simulink library "halin"  (R2021b)
settings: Solver=VariableStepAuto  StartTime=0.0  StopTime=10.0  RelTol=1e-3
undefined symbols (not defined in the file): TRUE
libraries: FVT_lib x100, hcu_lib x41
(part 3 of 10)

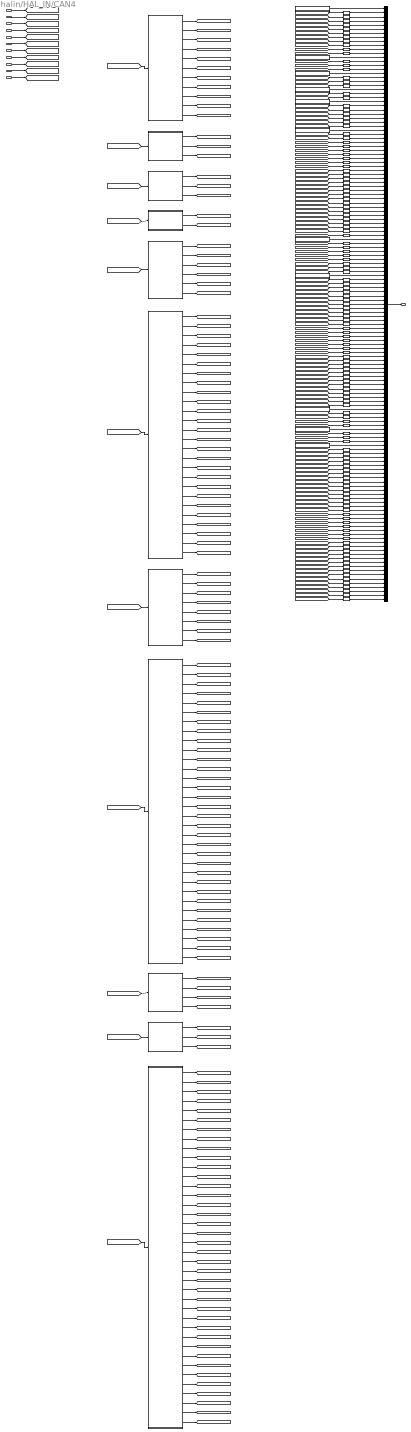
== system halin/HAL_IN/CAN4 ==
  DT_CAN4_SG_DKC1 : Inport
  DT_CAN4_SG_ZONE_DR_VCU : Inport  Port=2
  DT_CAN4_SG_ZONE_FR1 : Inport  Port=3
  DT_CAN4_SG_ZONE_FR_VCU : Inport  Port=4
  DT_CAN4_SG_zGW_APTC1 : Inport  Port=5
  DT_CAN4_SG_zGW_CANFr1 : Inport  Port=6
  DT_CAN4_SG_zGW_LINDr1 : Inport  Port=7
  DT_CAN4_SG_DKC2 : Inport  Port=8
  DT_CAN4_SG_Z24_C1000_0 : Inport  Port=9
  DT_CAN4_SG_Z24_CE100_0 : Inport  Port=10
  DT_CAN4_SG_ZONE_DR1 : Inport  Port=11
  DKC1 : Subsystem
  DKC2 : Subsystem
  UnitConverter{,1..7,9,25,31,33,35,37,39,41,43,45,47,49..50,58,60,62..67,70,72,74,76,78,80,82,84..88,90,99..100,102..104,120} (48 alike) : DataTypeConversion  OutDataTypeStr=uint8
  UnitConverter{8,10,17..20,23..24,26..29,51..52,55..57,68,98,101,105..107,109..110,112..113,115..116,118..119,121..135} (46 alike) : DataTypeConversion  OutDataTypeStr=boolean
  UnitConverter{14..16,21..22,30,32,34,36,38,40,42,44,46,48,53..54,59,61,69,71,73,75,77,79,81,83,89,91..96,108,111,114,117} (38 alike) : DataTypeConversion  OutDataTypeStr=single
  UnitConverter11 : DataTypeConversion  OutDataTypeStr=uint64
  UnitConverter12 : DataTypeConversion  OutDataTypeStr=uint64
  UnitConverter13 : DataTypeConversion  OutDataTypeStr=uint64
  UnitConverter97 : DataTypeConversion  OutDataTypeStr=uint16
  VHAL_CANMsgInvalidDKC1_flg : Subsystem  AncestorBlock=FVT_lib/hal/MsgTimeoutJudge_CAN_AUTOSAR
      mask help: MeasumentTrigerEvent
      mask Display: fprintf('MsgTimeoutJudge_CAN\nAUTOSAR');
  VHAL_CANMsgInvalidDKC2_flg : Subsystem  AncestorBlock=FVT_lib/hal/MsgTimeoutJudge_CAN_AUTOSAR
      mask help: MeasumentTrigerEvent
      mask Display: fprintf('MsgTimeoutJudge_CAN\nAUTOSAR');
  VHAL_CANMsgInvalidZ24C10000_flg : Subsystem  AncestorBlock=FVT_lib/hal/MsgTimeoutJudge_CAN_AUTOSAR
      mask help: MeasumentTrigerEvent
      mask Display: fprintf('MsgTimeoutJudge_CAN\nAUTOSAR');
  VHAL_CANMsgInvalidZ24CE1000_flg : Subsystem  AncestorBlock=FVT_lib/hal/MsgTimeoutJudge_CAN_AUTOSAR
      mask help: MeasumentTrigerEvent
      mask Display: fprintf('MsgTimeoutJudge_CAN\nAUTOSAR');
  VHAL_CANMsgInvalidZONEDR1_flg : Subsystem  AncestorBlock=FVT_lib/hal/MsgTimeoutJudge_CAN_AUTOSAR
      mask help: MeasumentTrigerEvent
      mask Display: fprintf('MsgTimeoutJudge_CAN\nAUTOSAR');
  VHAL_CANMsgInvalidZONEDRVCU_flg : Subsystem  AncestorBlock=FVT_lib/hal/MsgTimeoutJudge_CAN_AUTOSAR
      mask help: MeasumentTrigerEvent
      mask Display: fprintf('MsgTimeoutJudge_CAN\nAUTOSAR');
  VHAL_CANMsgInvalidZONEFR1_flg : Subsystem  AncestorBlock=FVT_lib/hal/MsgTimeoutJudge_CAN_AUTOSAR
      mask help: MeasumentTrigerEvent
      mask Display: fprintf('MsgTimeoutJudge_CAN\nAUTOSAR');
  VHAL_CANMsgInvalidZONEFRVCU_flg : Subsystem  AncestorBlock=FVT_lib/hal/MsgTimeoutJudge_CAN_AUTOSAR
      mask help: MeasumentTrigerEvent
      mask Display: fprintf('MsgTimeoutJudge_CAN\nAUTOSAR');
  VHAL_CANMsgInvalidzGWAPTC1_flg : Subsystem  AncestorBlock=FVT_lib/hal/MsgTimeoutJudge_CAN_AUTOSAR
      mask help: MeasumentTrigerEvent
      mask Display: fprintf('MsgTimeoutJudge_CAN\nAUTOSAR');
  VHAL_CANMsgInvalidzGWCANFr1_flg : Subsystem  AncestorBlock=FVT_lib/hal/MsgTimeoutJudge_CAN_AUTOSAR
      mask help: MeasumentTrigerEvent
      mask Display: fprintf('MsgTimeoutJudge_CAN\nAUTOSAR');
  VHAL_CANMsgInvalidzGWLINDr1_flg : Subsystem  AncestorBlock=FVT_lib/hal/MsgTimeoutJudge_CAN_AUTOSAR
      mask help: MeasumentTrigerEvent
      mask Display: fprintf('MsgTimeoutJudge_CAN\nAUTOSAR');
  Z24_C1000_0 : Subsystem
  Z24_CE100_0 : Subsystem
  ZONE_DR1 : Subsystem
  ZONE_DR_VCU : Subsystem
  ZONE_FR1 : Subsystem
  ZONE_FR_VCU : Subsystem
  bus_creator : BusCreator  Inputs=147
  zGW_APTC1 : Subsystem
  zGW_CANFr1 : Subsystem
  zGW_LINDr1 : Subsystem
  HAL_CAN4_outputs : Outport
  wires:
  DT_CAN4_SG_DKC1/1 -> [DT_CAN4_SG_DKC1]
  DT_CAN4_SG_ZONE_DR_VCU/1 -> [DT_CAN4_SG_ZONE_DR_VCU]
  DT_CAN4_SG_ZONE_FR1/1 -> [DT_CAN4_SG_ZONE_FR1]
  DT_CAN4_SG_ZONE_FR_VCU/1 -> [DT_CAN4_SG_ZONE_FR_VCU]
  DT_CAN4_SG_zGW_APTC1/1 -> [DT_CAN4_SG_zGW_APTC1]
  DT_CAN4_SG_zGW_CANFr1/1 -> [DT_CAN4_SG_zGW_CANFr1]
  DT_CAN4_SG_zGW_LINDr1/1 -> [DT_CAN4_SG_zGW_LINDr1]
  DT_CAN4_SG_DKC2/1 -> [DT_CAN4_SG_DKC2]
  DT_CAN4_SG_Z24_C1000_0/1 -> [DT_CAN4_SG_Z24_C1000_0]
  DT_CAN4_SG_Z24_CE100_0/1 -> [DT_CAN4_SG_Z24_CE100_0]
  DT_CAN4_SG_ZONE_DR1/1 -> [DT_CAN4_SG_ZONE_DR1]
  [DT_CAN4_SG_DKC1] -> DKC1/1(DT_CAN4_SG_DKC1)
  [DT_CAN4_SG_DKC2] -> DKC2/1(DT_CAN4_SG_DKC2)
  [DT_CAN4_SG_Z24_C1000_0] -> Z24_C1000_0/1(DT_CAN4_SG_Z24_C1000_0)
  [DT_CAN4_SG_Z24_CE100_0] -> Z24_CE100_0/1(DT_CAN4_SG_Z24_CE100_0)
  [DT_CAN4_SG_ZONE_DR1] -> ZONE_DR1/1(DT_CAN4_SG_ZONE_DR1)
  [DT_CAN4_SG_ZONE_DR_VCU] -> ZONE_DR_VCU/1(DT_CAN4_SG_ZONE_DR_VCU)
  [DT_CAN4_SG_ZONE_FR1] -> ZONE_FR1/1(DT_CAN4_SG_ZONE_FR1)
  [DT_CAN4_SG_ZONE_FR_VCU] -> ZONE_FR_VCU/1(DT_CAN4_SG_ZONE_FR_VCU)
  [DT_CAN4_SG_zGW_APTC1] -> zGW_APTC1/1(DT_CAN4_SG_zGW_APTC1)
  [DT_CAN4_SG_zGW_CANFr1] -> zGW_CANFr1/1(DT_CAN4_SG_zGW_CANFr1)
  [DT_CAN4_SG_zGW_LINDr1] -> zGW_LINDr1/1(DT_CAN4_SG_zGW_LINDr1)
  bus_creator/1 -> HAL_CAN4_outputs/1
  VHAL_CANMsgInvalidDKC1_flg/1(Out) -> bus_creator/1
  DKC1/1(VHAL_DKCReVehData_enum) -> [VHAL_DKCReVehData_enum]
  UnitConverter/1 -> bus_creator/2  "VHAL_DKCReVehData_enum"
  [VHAL_DKCReVehData_enum] -> UnitConverter/1
  DKC1/2(VHAL_PCommandToBCM_enum) -> [VHAL_PCommandToBCM_enum]
  UnitConverter1/1 -> bus_creator/3  "VHAL_PCommandToBCM_enum"
  [VHAL_PCommandToBCM_enum] -> UnitConverter1/1
  DKC1/3(VHAL_PCommandToPTG_enum) -> [VHAL_PCommandToPTG_enum]
  UnitConverter2/1 -> bus_creator/4  "VHAL_PCommandToPTG_enum"
  [VHAL_PCommandToPTG_enum] -> UnitConverter2/1
  DKC1/4(VHAL_PDKeyAreaLockUnlock_enum) -> [VHAL_PDKeyAreaLockUnlock_enum]
  UnitConverter3/1 -> bus_creator/5  "VHAL_PDKeyAreaLockUnlock_enum"
  [VHAL_PDKeyAreaLockUnlock_enum] -> UnitConverter3/1
  DKC1/5(VHAL_PDKeyAreaPS_enum) -> [VHAL_PDKeyAreaPS_enum]
  UnitConverter4/1 -> bus_creator/6  "VHAL_PDKeyAreaPS_enum"
  [VHAL_PDKeyAreaPS_enum] -> UnitConverter4/1
  DKC1/6(VHAL_PDKeyAreaPTG_enum) -> [VHAL_PDKeyAreaPTG_enum]
  UnitConverter5/1 -> bus_creator/7  "VHAL_PDKeyAreaPTG_enum"
  [VHAL_PDKeyAreaPTG_enum] -> UnitConverter5/1
  DKC1/7(VHAL_PDKeyWelcome_enum) -> [VHAL_PDKeyWelcome_enum]
  UnitConverter6/1 -> bus_creator/8  "VHAL_PDKeyWelcome_enum"
  [VHAL_PDKeyWelcome_enum] -> UnitConverter6/1
  DKC1/8(VHAL_PDkeyShowIVI_enum) -> [VHAL_PDkeyShowIVI_enum]
  UnitConverter7/1 -> bus_creator/9  "VHAL_PDkeyShowIVI_enum"
  [VHAL_PDkeyShowIVI_enum] -> UnitConverter7/1
  DKC1/9(VHAL_PKeyMiss_flg) -> [VHAL_PKeyMiss_flg]
  UnitConverter8/1 -> bus_creator/10  "VHAL_PKeyMiss_flg"
  [VHAL_PKeyMiss_flg] -> UnitConverter8/1
  DKC1/10(VHAL_PKeyMode_enum) -> [VHAL_PKeyMode_enum]
  UnitConverter9/1 -> bus_creator/11  "VHAL_PKeyMode_enum"
  [VHAL_PKeyMode_enum] -> UnitConverter9/1
  DKC1/11(VHAL_PUIDLowPower_flg) -> [VHAL_PUIDLowPower_flg]
  UnitConverter10/1 -> bus_creator/12  "VHAL_PUIDLowPower_flg"
  [VHAL_PUIDLowPower_flg] -> UnitConverter10/1
  VHAL_CANMsgInvalidDKC2_flg/1(Out) -> bus_creator/13
  DKC2/1(VHAL_EncryptionDATA063_enum) -> [VHAL_EncryptionDATA063_enum]
  UnitConverter11/1 -> bus_creator/14  "VHAL_EncryptionDATA063_enum"
  [VHAL_EncryptionDATA063_enum] -> UnitConverter11/1
  DKC2/2(VHAL_EncryptionDATA64127_enum) -> [VHAL_EncryptionDATA64127_enum]
  UnitConverter12/1 -> bus_creator/15  "VHAL_EncryptionDATA64127_enum"
  [VHAL_EncryptionDATA64127_enum] -> UnitConverter12/1
  DKC2/3(VHAL_RandomNumberX_enum) -> [VHAL_RandomNumberX_enum]
  UnitConverter13/1 -> bus_creator/16  "VHAL_RandomNumberX_enum"
  [VHAL_RandomNumberX_enum] -> UnitConverter13/1
  VHAL_CANMsgInvalidZ24C10000_flg/1(Out) -> bus_creator/17
  Z24_C1000_0/1(VHAL_Z24CHAAirPressureFC2Sta_KPa) -> [VHAL_Z24CHAAirPressureFC2Sta_KPa]
  UnitConverter14/1 -> bus_creator/18  "VHAL_Z24CHAAirPressureFC2Sta_KPa"
  [VHAL_Z24CHAAirPressureFC2Sta_KPa] -> UnitConverter14/1
  Z24_C1000_0/2(VHAL_Z24CHAAirPressurePC3Sta_KPa) -> [VHAL_Z24CHAAirPressurePC3Sta_KPa]
  UnitConverter15/1 -> bus_creator/19  "VHAL_Z24CHAAirPressurePC3Sta_KPa"
  [VHAL_Z24CHAAirPressurePC3Sta_KPa] -> UnitConverter15/1
  Z24_C1000_0/3(VHAL_Z24CHAAirPressureRC1Sta_KPa) -> [VHAL_Z24CHAAirPressureRC1Sta_KPa]
  UnitConverter16/1 -> bus_creator/20  "VHAL_Z24CHAAirPressureRC1Sta_KPa"
  [VHAL_Z24CHAAirPressureRC1Sta_KPa] -> UnitConverter16/1
  VHAL_CANMsgInvalidZ24CE1000_flg/1(Out) -> bus_creator/21
  Z24_CE100_0/1(VHAL_Z24BCMFWiperASSta_flg) -> [VHAL_Z24BCMFWiperASSta_flg]
  UnitConverter17/1 -> bus_creator/22  "VHAL_Z24BCMFWiperASSta_flg"
  [VHAL_Z24BCMFWiperASSta_flg] -> UnitConverter17/1
  Z24_CE100_0/2(VHAL_Z24BCMSeatBeltSWSta_flg) -> [VHAL_Z24BCMSeatBeltSWSta_flg]
  UnitConverter18/1 -> bus_creator/23  "VHAL_Z24BCMSeatBeltSWSta_flg"
  [VHAL_Z24BCMSeatBeltSWSta_flg] -> UnitConverter18/1
  VHAL_CANMsgInvalidZONEDR1_flg/1(Out) -> bus_creator/24
  ZONE_DR1/1(VHAL_DrLockSta_flg) -> [VHAL_DrLockSta_flg]
  UnitConverter19/1 -> bus_creator/25  "VHAL_DrLockSta_flg"
  [VHAL_DrLockSta_flg] -> UnitConverter19/1
  ZONE_DR1/2(VHAL_MIRRORFOLDSW_flg) -> [VHAL_MIRRORFOLDSW_flg]
  UnitConverter20/1 -> bus_creator/26  "VHAL_MIRRORFOLDSW_flg"
  [VHAL_MIRRORFOLDSW_flg] -> UnitConverter20/1
  ZONE_DR1/3(VHAL_RLTurnLampC_mA) -> [VHAL_RLTurnLampC_mA]
  UnitConverter21/1 -> bus_creator/27  "VHAL_RLTurnLampC_mA"
  [VHAL_RLTurnLampC_mA] -> UnitConverter21/1
  ZONE_DR1/4(VHAL_RRTurnLampC_mA) -> [VHAL_RRTurnLampC_mA]
  UnitConverter22/1 -> bus_creator/28  "VHAL_RRTurnLampC_mA"
  [VHAL_RRTurnLampC_mA] -> UnitConverter22/1
  ZONE_DR1/5(VHAL_RWiperAS_flg) -> [VHAL_RWiperAS_flg]
  UnitConverter23/1 -> bus_creator/29  "VHAL_RWiperAS_flg"
  [VHAL_RWiperAS_flg] -> UnitConverter23/1
  ZONE_DR1/6(VHAL_RWiperProtection_flg) -> [VHAL_RWiperProtection_flg]
  UnitConverter24/1 -> bus_creator/30  "VHAL_RWiperProtection_flg"
  [VHAL_RWiperProtection_flg] -> UnitConverter24/1
  VHAL_CANMsgInvalidZONEDRVCU_flg/1(Out) -> bus_creator/31
  ZONE_DR_VCU/1(VHAL_BlowerErr_enum) -> [VHAL_BlowerErr_enum]
  UnitConverter25/1 -> bus_creator/32  "VHAL_BlowerErr_enum"
  [VHAL_BlowerErr_enum] -> UnitConverter25/1
  ZONE_DR_VCU/2(VHAL_DrPMMLVOutPErrLmp_flg) -> [VHAL_DrPMMLVOutPErrLmp_flg]
  UnitConverter26/1 -> bus_creator/33  "VHAL_DrPMMLVOutPErrLmp_flg"
  [VHAL_DrPMMLVOutPErrLmp_flg] -> UnitConverter26/1
  ZONE_DR_VCU/3(VHAL_DrPMMSysErrLmp_flg) -> [VHAL_DrPMMSysErrLmp_flg]
  UnitConverter27/1 -> bus_creator/34  "VHAL_DrPMMSysErrLmp_flg"
  [VHAL_DrPMMSysErrLmp_flg] -> UnitConverter27/1
  ZONE_DR_VCU/4(VHAL_DrSCPSysErrLmp_flg) -> [VHAL_DrSCPSysErrLmp_flg]
  UnitConverter28/1 -> bus_creator/35  "VHAL_DrSCPSysErrLmp_flg"
  [VHAL_DrSCPSysErrLmp_flg] -> UnitConverter28/1
  ZONE_DR_VCU/5(VHAL_DrStdAErrSta_flg) -> [VHAL_DrStdAErrSta_flg]
  UnitConverter29/1 -> bus_creator/36  "VHAL_DrStdAErrSta_flg"
  [VHAL_DrStdAErrSta_flg] -> UnitConverter29/1
  ZONE_DR_VCU/6(VHAL_SolarL_W) -> [VHAL_SolarL_W]
  UnitConverter30/1 -> bus_creator/37  "VHAL_SolarL_W"
  [VHAL_SolarL_W] -> UnitConverter30/1
  ZONE_DR_VCU/7(VHAL_SolarLErr_enum) -> [VHAL_SolarLErr_enum]
  UnitConverter31/1 -> bus_creator/38  "VHAL_SolarLErr_enum"
  [VHAL_SolarLErr_enum] -> UnitConverter31/1
  ZONE_DR_VCU/8(VHAL_SolarR_W) -> [VHAL_SolarR_W]
  UnitConverter32/1 -> bus_creator/39  "VHAL_SolarR_W"
  [VHAL_SolarR_W] -> UnitConverter32/1
  ZONE_DR_VCU/9(VHAL_SolarRErr_enum) -> [VHAL_SolarRErr_enum]
  UnitConverter33/1 -> bus_creator/40  "VHAL_SolarRErr_enum"
  [VHAL_SolarRErr_enum] -> UnitConverter33/1
  ZONE_DR_VCU/10(VHAL_TFaceL_C) -> [VHAL_TFaceL_C]
  UnitConverter34/1 -> bus_creator/41  "VHAL_TFaceL_C"
  [VHAL_TFaceL_C] -> UnitConverter34/1
  ZONE_DR_VCU/11(VHAL_TFaceLErr_enum) -> [VHAL_TFaceLErr_enum]
  UnitConverter35/1 -> bus_creator/42  "VHAL_TFaceLErr_enum"
  [VHAL_TFaceLErr_enum] -> UnitConverter35/1
  ZONE_DR_VCU/12(VHAL_TFaceR_C) -> [VHAL_TFaceR_C]
  UnitConverter36/1 -> bus_creator/43  "VHAL_TFaceR_C"
  [VHAL_TFaceR_C] -> UnitConverter36/1
  ZONE_DR_VCU/13(VHAL_TFaceRErr_enum) -> [VHAL_TFaceRErr_enum]
  UnitConverter37/1 -> bus_creator/44  "VHAL_TFaceRErr_enum"
  [VHAL_TFaceRErr_enum] -> UnitConverter37/1
  ZONE_DR_VCU/14(VHAL_TFaceRr_C) -> [VHAL_TFaceRr_C]
  UnitConverter38/1 -> bus_creator/45  "VHAL_TFaceRr_C"
  [VHAL_TFaceRr_C] -> UnitConverter38/1
  ZONE_DR_VCU/15(VHAL_TFaceRrErr_enum) -> [VHAL_TFaceRrErr_enum]
  UnitConverter39/1 -> bus_creator/46  "VHAL_TFaceRrErr_enum"
  [VHAL_TFaceRrErr_enum] -> UnitConverter39/1
  ZONE_DR_VCU/16(VHAL_TFootL_C) -> [VHAL_TFootL_C]
  UnitConverter40/1 -> bus_creator/47  "VHAL_TFootL_C"
  [VHAL_TFootL_C] -> UnitConverter40/1
  ZONE_DR_VCU/17(VHAL_TFootLErr_enum) -> [VHAL_TFootLErr_enum]
  UnitConverter41/1 -> bus_creator/48  "VHAL_TFootLErr_enum"
  [VHAL_TFootLErr_enum] -> UnitConverter41/1
  ZONE_DR_VCU/18(VHAL_TFootR_C) -> [VHAL_TFootR_C]
  UnitConverter42/1 -> bus_creator/49  "VHAL_TFootR_C"
  [VHAL_TFootR_C] -> UnitConverter42/1
  ZONE_DR_VCU/19(VHAL_TFootRErr_enum) -> [VHAL_TFootRErr_enum]
  UnitConverter43/1 -> bus_creator/50  "VHAL_TFootRErr_enum"
  [VHAL_TFootRErr_enum] -> UnitConverter43/1
  ZONE_DR_VCU/20(VHAL_TFootRr_C) -> [VHAL_TFootRr_C]
  UnitConverter44/1 -> bus_creator/51  "VHAL_TFootRr_C"
  [VHAL_TFootRr_C] -> UnitConverter44/1
  ZONE_DR_VCU/21(VHAL_TFootRrErr_enum) -> [VHAL_TFootRrErr_enum]
  UnitConverter45/1 -> bus_creator/52  "VHAL_TFootRrErr_enum"
  [VHAL_TFootRrErr_enum] -> UnitConverter45/1
  ZONE_DR_VCU/22(VHAL_Tevap_C) -> [VHAL_Tevap_C]
  UnitConverter46/1 -> bus_creator/53  "VHAL_Tevap_C"
  [VHAL_Tevap_C] -> UnitConverter46/1
  ZONE_DR_VCU/23(VHAL_TevapErr_enum) -> [VHAL_TevapErr_enum]
  UnitConverter47/1 -> bus_creator/54  "VHAL_TevapErr_enum"
  [VHAL_TevapErr_enum] -> UnitConverter47/1
  ZONE_DR_VCU/24(VHAL_Tincar_C) -> [VHAL_Tincar_C]
  UnitConverter48/1 -> bus_creator/55  "VHAL_Tincar_C"
  [VHAL_Tincar_C] -> UnitConverter48/1
  ZONE_DR_VCU/25(VHAL_TincarErr_enum) -> [VHAL_TincarErr_enum]
  UnitConverter49/1 -> bus_creator/56  "VHAL_TincarErr_enum"
  [VHAL_TincarErr_enum] -> UnitConverter49/1
  ZONE_DR_VCU/26(VHAL_ZoneDrMalfunLevel_enum) -> [VHAL_ZoneDrMalfunLevel_enum]
  UnitConverter50/1 -> bus_creator/57  "VHAL_ZoneDrMalfunLevel_enum"
  [VHAL_ZoneDrMalfunLevel_enum] -> UnitConverter50/1
  VHAL_CANMsgInvalidZONEFR1_flg/1(Out) -> bus_creator/58
  ZONE_FR1/1(VHAL_ChargeInletLockSta_flg) -> [VHAL_ChargeInletLockSta_flg]
  UnitConverter51/1 -> bus_creator/59  "VHAL_ChargeInletLockSta_flg"
  [VHAL_ChargeInletLockSta_flg] -> UnitConverter51/1
  ZONE_FR1/2(VHAL_CompProEN_flg) -> [VHAL_CompProEN_flg]
  UnitConverter52/1 -> bus_creator/60  "VHAL_CompProEN_flg"
  [VHAL_CompProEN_flg] -> UnitConverter52/1
  ZONE_FR1/3(VHAL_FLTurnLampC_mA) -> [VHAL_FLTurnLampC_mA]
  UnitConverter53/1 -> bus_creator/61  "VHAL_FLTurnLampC_mA"
  [VHAL_FLTurnLampC_mA] -> UnitConverter53/1
  ZONE_FR1/4(VHAL_FRTurnLampC_mA) -> [VHAL_FRTurnLampC_mA]
  UnitConverter54/1 -> bus_creator/62  "VHAL_FRTurnLampC_mA"
  [VHAL_FRTurnLampC_mA] -> UnitConverter54/1
  ZONE_FR1/5(VHAL_FWiperAS_flg) -> [VHAL_FWiperAS_flg]
  UnitConverter55/1 -> bus_creator/63  "VHAL_FWiperAS_flg"
  [VHAL_FWiperAS_flg] -> UnitConverter55/1
  ZONE_FR1/6(VHAL_FWiperProtection_flg) -> [VHAL_FWiperProtection_flg]
  UnitConverter56/1 -> bus_creator/64  "VHAL_FWiperProtection_flg"
  [VHAL_FWiperProtection_flg] -> UnitConverter56/1
  ZONE_FR1/7(VHAL_TrailerCheck_flg) -> [VHAL_TrailerCheck_flg]
  UnitConverter57/1 -> bus_creator/65  "VHAL_TrailerCheck_flg"
  [VHAL_TrailerCheck_flg] -> UnitConverter57/1
  ZONE_FR1/8(VHAL_TrailerModeSta_enum) -> [VHAL_TrailerModeSta_enum]
  UnitConverter58/1 -> bus_creator/66  "VHAL_TrailerModeSta_enum"
  [VHAL_TrailerModeSta_enum] -> UnitConverter58/1
  VHAL_CANMsgInvalidZONEFRVCU_flg/1(Out) -> bus_creator/67
  ZONE_FR_VCU/1(VHAL_BatInTemp_C) -> [VHAL_BatInTemp_C]
  UnitConverter59/1 -> bus_creator/68  "VHAL_BatInTemp_C"
  [VHAL_BatInTemp_C] -> UnitConverter59/1
  ZONE_FR_VCU/2(VHAL_BatInTempErr_enum) -> [VHAL_BatInTempErr_enum]
  UnitConverter60/1 -> bus_creator/69  "VHAL_BatInTempErr_enum"
  [VHAL_BatInTempErr_enum] -> UnitConverter60/1
  ZONE_FR_VCU/3(VHAL_BatOutTemp_C) -> [VHAL_BatOutTemp_C]
  UnitConverter61/1 -> bus_creator/70  "VHAL_BatOutTemp_C"
  [VHAL_BatOutTemp_C] -> UnitConverter61/1
  ZONE_FR_VCU/4(VHAL_COMPErr_enum) -> [VHAL_COMPErr_enum]
  UnitConverter62/1 -> bus_creator/71  "VHAL_COMPErr_enum"
  [VHAL_COMPErr_enum] -> UnitConverter62/1
  ZONE_FR_VCU/5(VHAL_EACProtectEnable_enum) -> [VHAL_EACProtectEnable_enum]
  UnitConverter63/1 -> bus_creator/72  "VHAL_EACProtectEnable_enum"
  [VHAL_EACProtectEnable_enum] -> UnitConverter63/1
  ZONE_FR_VCU/6(VHAL_EWP3Err_enum) -> [VHAL_EWP3Err_enum]
  UnitConverter64/1 -> bus_creator/73  "VHAL_EWP3Err_enum"
  [VHAL_EWP3Err_enum] -> UnitConverter64/1
  ZONE_FR_VCU/7(VHAL_EXV1Err_enum) -> [VHAL_EXV1Err_enum]
  UnitConverter65/1 -> bus_creator/74  "VHAL_EXV1Err_enum"
  [VHAL_EXV1Err_enum] -> UnitConverter65/1
  ZONE_FR_VCU/8(VHAL_EXV2Err_enum) -> [VHAL_EXV2Err_enum]
  UnitConverter66/1 -> bus_creator/75  "VHAL_EXV2Err_enum"
  [VHAL_EXV2Err_enum] -> UnitConverter66/1
  ZONE_FR_VCU/9(VHAL_FanErr_enum) -> [VHAL_FanErr_enum]
  UnitConverter67/1 -> bus_creator/76  "VHAL_FanErr_enum"
  [VHAL_FanErr_enum] -> UnitConverter67/1
  ZONE_FR_VCU/10(VHAL_FrPMMLimpHomeActReq_flg) -> [VHAL_FrPMMLimpHomeActReq_flg]
  UnitConverter68/1 -> bus_creator/77  "VHAL_FrPMMLimpHomeActReq_flg"
  [VHAL_FrPMMLimpHomeActReq_flg] -> UnitConverter68/1
  ZONE_FR_VCU/11(VHAL_MotorInTemp_C) -> [VHAL_MotorInTemp_C]
  UnitConverter69/1 -> bus_creator/78  "VHAL_MotorInTemp_C"
  [VHAL_MotorInTemp_C] -> UnitConverter69/1
  ZONE_FR_VCU/12(VHAL_MotorInTempErr_enum) -> [VHAL_MotorInTempErr_enum]
  UnitConverter70/1 -> bus_creator/79  "VHAL_MotorInTempErr_enum"
  [VHAL_MotorInTempErr_enum] -> UnitConverter70/1
  ZONE_FR_VCU/13(VHAL_MotorOutTemp_C) -> [VHAL_MotorOutTemp_C]
  UnitConverter71/1 -> bus_creator/80  "VHAL_MotorOutTemp_C"
  [VHAL_MotorOutTemp_C] -> UnitConverter71/1
  ZONE_FR_VCU/14(VHAL_MotorOutTempErr_enum) -> [VHAL_MotorOutTempErr_enum]
  UnitConverter72/1 -> bus_creator/81  "VHAL_MotorOutTempErr_enum"
  [VHAL_MotorOutTempErr_enum] -> UnitConverter72/1
  ZONE_FR_VCU/15(VHAL_PTHighP_KPa) -> [VHAL_PTHighP_KPa]
  UnitConverter73/1 -> bus_creator/82  "VHAL_PTHighP_KPa"
  [VHAL_PTHighP_KPa] -> UnitConverter73/1
  ZONE_FR_VCU/16(VHAL_PTHighPErr_enum) -> [VHAL_PTHighPErr_enum]
  UnitConverter74/1 -> bus_creator/83  "VHAL_PTHighPErr_enum"
  [VHAL_PTHighPErr_enum] -> UnitConverter74/1
  ZONE_FR_VCU/17(VHAL_PTHighTact_C) -> [VHAL_PTHighTact_C]
  UnitConverter75/1 -> bus_creator/84  "VHAL_PTHighTact_C"
  [VHAL_PTHighTact_C] -> UnitConverter75/1
  ZONE_FR_VCU/18(VHAL_PTHighTactErr_enum) -> [VHAL_PTHighTactErr_enum]
  UnitConverter76/1 -> bus_creator/85  "VHAL_PTHighTactErr_enum"
  [VHAL_PTHighTactErr_enum] -> UnitConverter76/1
  ZONE_FR_VCU/19(VHAL_PTLowP1_KPa) -> [VHAL_PTLowP1_KPa]
  UnitConverter77/1 -> bus_creator/86  "VHAL_PTLowP1_KPa"
  [VHAL_PTLowP1_KPa] -> UnitConverter77/1
  ZONE_FR_VCU/20(VHAL_PTLowP1Err_enum) -> [VHAL_PTLowP1Err_enum]
  UnitConverter78/1 -> bus_creator/87  "VHAL_PTLowP1Err_enum"
  [VHAL_PTLowP1Err_enum] -> UnitConverter78/1
  ZONE_FR_VCU/21(VHAL_PTLowP2_KPa) -> [VHAL_PTLowP2_KPa]
  UnitConverter79/1 -> bus_creator/88  "VHAL_PTLowP2_KPa"
  [VHAL_PTLowP2_KPa] -> UnitConverter79/1
  ZONE_FR_VCU/22(VHAL_PTLowP2Err_enum) -> [VHAL_PTLowP2Err_enum]
  UnitConverter80/1 -> bus_creator/89  "VHAL_PTLowP2Err_enum"
  [VHAL_PTLowP2Err_enum] -> UnitConverter80/1
  ZONE_FR_VCU/23(VHAL_PTLowT1_C) -> [VHAL_PTLowT1_C]
  UnitConverter81/1 -> bus_creator/90  "VHAL_PTLowT1_C"
  [VHAL_PTLowT1_C] -> UnitConverter81/1
  ZONE_FR_VCU/24(VHAL_PTLowT1Err_enum) -> [VHAL_PTLowT1Err_enum]
  UnitConverter82/1 -> bus_creator/91  "VHAL_PTLowT1Err_enum"
  [VHAL_PTLowT1Err_enum] -> UnitConverter82/1
  ZONE_FR_VCU/25(VHAL_PTLowT2_C) -> [VHAL_PTLowT2_C]
  UnitConverter83/1 -> bus_creator/92  "VHAL_PTLowT2_C"
  [VHAL_PTLowT2_C] -> UnitConverter83/1
  ZONE_FR_VCU/26(VHAL_PTLowT2Err_enum) -> [VHAL_PTLowT2Err_enum]
  UnitConverter84/1 -> bus_creator/93  "VHAL_PTLowT2Err_enum"
  [VHAL_PTLowT2Err_enum] -> UnitConverter84/1
  ZONE_FR_VCU/27(VHAL_SOTXVErr_enum) -> [VHAL_SOTXVErr_enum]
  UnitConverter85/1 -> bus_creator/94  "VHAL_SOTXVErr_enum"
  [VHAL_SOTXVErr_enum] -> UnitConverter85/1
  ZONE_FR_VCU/28(VHAL_SOV1Err_enum) -> [VHAL_SOV1Err_enum]
  UnitConverter86/1 -> bus_creator/95  "VHAL_SOV1Err_enum"
  [VHAL_SOV1Err_enum] -> UnitConverter86/1
  ZONE_FR_VCU/29(VHAL_SOV2Err_enum) -> [VHAL_SOV2Err_enum]
  UnitConverter87/1 -> bus_creator/96  "VHAL_SOV2Err_enum"
  [VHAL_SOV2Err_enum] -> UnitConverter87/1
  ZONE_FR_VCU/30(VHAL_SOV3Err_enum) -> [VHAL_SOV3Err_enum]
  UnitConverter88/1 -> bus_creator/97  "VHAL_SOV3Err_enum"
  [VHAL_SOV3Err_enum] -> UnitConverter88/1
  ZONE_FR_VCU/31(VHAL_Tamb_C) -> [VHAL_Tamb_C]
  UnitConverter89/1 -> bus_creator/98  "VHAL_Tamb_C"
  [VHAL_Tamb_C] -> UnitConverter89/1
  ZONE_FR_VCU/32(VHAL_TambErr_enum) -> [VHAL_TambErr_enum]
  UnitConverter90/1 -> bus_creator/99  "VHAL_TambErr_enum"
  [VHAL_TambErr_enum] -> UnitConverter90/1
  VHAL_CANMsgInvalidzGWAPTC1_flg/1(Out) -> bus_creator/100
  zGW_APTC1/1(VHAL_FrntPTCLeActHeatPwr_W) -> [VHAL_FrntPTCLeActHeatPwr_W]
  UnitConverter91/1 -> bus_creator/101  "VHAL_FrntPTCLeActHeatPwr_W"
  [VHAL_FrntPTCLeActHeatPwr_W] -> UnitConverter91/1
  zGW_APTC1/2(VHAL_FrntPTCRearLeActHeatPwr_W) -> [VHAL_FrntPTCRearLeActHeatPwr_W]
  UnitConverter92/1 -> bus_creator/102  "VHAL_FrntPTCRearLeActHeatPwr_W"
  [VHAL_FrntPTCRearLeActHeatPwr_W] -> UnitConverter92/1
  zGW_APTC1/3(VHAL_FrntPTCRearRiActHeatPwr_W) -> [VHAL_FrntPTCRearRiActHeatPwr_W]
  UnitConverter93/1 -> bus_creator/103  "VHAL_FrntPTCRearRiActHeatPwr_W"
  [VHAL_FrntPTCRearRiActHeatPwr_W] -> UnitConverter93/1
  zGW_APTC1/4(VHAL_FrntPTCRiActHeatPwr_W) -> [VHAL_FrntPTCRiActHeatPwr_W]
  UnitConverter94/1 -> bus_creator/104  "VHAL_FrntPTCRiActHeatPwr_W"
  [VHAL_FrntPTCRiActHeatPwr_W] -> UnitConverter94/1
  VHAL_CANMsgInvalidzGWCANFr1_flg/1(Out) -> bus_creator/105
  zGW_CANFr1/1(VHAL_COMPActualPwr_W) -> [VHAL_COMPActualPwr_W]
  UnitConverter95/1 -> bus_creator/106  "VHAL_COMPActualPwr_W"
  [VHAL_COMPActualPwr_W] -> UnitConverter95/1
  zGW_CANFr1/2(VHAL_COMPStatorSpd_rpm) -> [VHAL_COMPStatorSpd_rpm]
  UnitConverter96/1 -> bus_creator/107  "VHAL_COMPStatorSpd_rpm"
  [VHAL_COMPStatorSpd_rpm] -> UnitConverter96/1
  zGW_CANFr1/3(VHAL_PTCActuPwrHSC6_enum) -> [VHAL_PTCActuPwrHSC6_enum]
  UnitConverter97/1 -> bus_creator/108  "VHAL_PTCActuPwrHSC6_enum"
  [VHAL_PTCActuPwrHSC6_enum] -> UnitConverter97/1
  VHAL_CANMsgInvalidzGWLINDr1_flg/1(Out) -> bus_creator/109
  zGW_LINDr1/1(VHAL_CSWDimSw_flg) -> [VHAL_CSWDimSw_flg]
  UnitConverter98/1 -> bus_creator/110  "VHAL_CSWDimSw_flg"
  [VHAL_CSWDimSw_flg] -> UnitConverter98/1
  zGW_LINDr1/2(VHAL_CSWFWasSwSta_enum) -> [VHAL_CSWFWasSwSta_enum]
  UnitConverter99/1 -> bus_creator/111  "VHAL_CSWFWasSwSta_enum"
  [VHAL_CSWFWasSwSta_enum] -> UnitConverter99/1
  zGW_LINDr1/3(VHAL_CSWFWipSwSta_enum) -> [VHAL_CSWFWipSwSta_enum]
  UnitConverter100/1 -> bus_creator/112  "VHAL_CSWFWipSwSta_enum"
  [VHAL_CSWFWipSwSta_enum] -> UnitConverter100/1
  zGW_LINDr1/4(VHAL_CSWPassSWSta_flg) -> [VHAL_CSWPassSWSta_flg]
  UnitConverter101/1 -> bus_creator/113  "VHAL_CSWPassSWSta_flg"
  [VHAL_CSWPassSWSta_flg] -> UnitConverter101/1
  zGW_LINDr1/5(VHAL_CSWRWasSWSta_enum) -> [VHAL_CSWRWasSWSta_enum]
  UnitConverter102/1 -> bus_creator/114  "VHAL_CSWRWasSWSta_enum"
  [VHAL_CSWRWasSWSta_enum] -> UnitConverter102/1
  zGW_LINDr1/6(VHAL_CSWRWipIntSwSta_enum) -> [VHAL_CSWRWipIntSwSta_enum]
  UnitConverter103/1 -> bus_creator/115  "VHAL_CSWRWipIntSwSta_enum"
  [VHAL_CSWRWipIntSwSta_enum] -> UnitConverter103/1
  zGW_LINDr1/7(VHAL_CSWTurnSwSta_enum) -> [VHAL_CSWTurnSwSta_enum]
  UnitConverter104/1 -> bus_creator/116  "VHAL_CSWTurnSwSta_enum"
  [VHAL_CSWTurnSwSta_enum] -> UnitConverter104/1
  zGW_LINDr1/8(VHAL_FAPWL01LINResponseError_flg) -> [VHAL_FAPWL01LINResponseError_flg]
  UnitConverter105/1 -> bus_creator/117  "VHAL_FAPWL01LINResponseError_flg"
  [VHAL_FAPWL01LINResponseError_flg] -> UnitConverter105/1
  zGW_LINDr1/9(VHAL_LDrvMotorRelayError_flg) -> [VHAL_LDrvMotorRelayError_flg]
  UnitConverter106/1 -> bus_creator/118  "VHAL_LDrvMotorRelayError_flg"
  [VHAL_LDrvMotorRelayError_flg] -> UnitConverter106/1
  zGW_LINDr1/10(VHAL_LDrvMotorRippleError_flg) -> [VHAL_LDrvMotorRippleError_flg]
  UnitConverter107/1 -> bus_creator/119  "VHAL_LDrvMotorRippleError_flg"
  [VHAL_LDrvMotorRippleError_flg] -> UnitConverter107/1
  zGW_LINDr1/11(VHAL_LDrvValWdwOpened_pct) -> [VHAL_LDrvValWdwOpened_pct]
  UnitConverter108/1 -> bus_creator/120  "VHAL_LDrvValWdwOpened_pct"
  [VHAL_LDrvValWdwOpened_pct] -> UnitConverter108/1
  zGW_LINDr1/12(VHAL_LPasMotorRelayError_flg) -> [VHAL_LPasMotorRelayError_flg]
  UnitConverter109/1 -> bus_creator/121  "VHAL_LPasMotorRelayError_flg"
  [VHAL_LPasMotorRelayError_flg] -> UnitConverter109/1
  zGW_LINDr1/13(VHAL_LPasMotorRippleError_flg) -> [VHAL_LPasMotorRippleError_flg]
  UnitConverter110/1 -> bus_creator/122  "VHAL_LPasMotorRippleError_flg"
  [VHAL_LPasMotorRippleError_flg] -> UnitConverter110/1
  zGW_LINDr1/14(VHAL_LPasValWdwOpened_pct) -> [VHAL_LPasValWdwOpened_pct]
  UnitConverter111/1 -> bus_creator/123  "VHAL_LPasValWdwOpened_pct"
  [VHAL_LPasValWdwOpened_pct] -> UnitConverter111/1
  zGW_LINDr1/15(VHAL_LRLDMotorRelayError_flg) -> [VHAL_LRLDMotorRelayError_flg]
  UnitConverter112/1 -> bus_creator/124  "VHAL_LRLDMotorRelayError_flg"
  [VHAL_LRLDMotorRelayError_flg] -> UnitConverter112/1
  zGW_LINDr1/16(VHAL_LRLDMotorRippleError_flg) -> [VHAL_LRLDMotorRippleError_flg]
  UnitConverter113/1 -> bus_creator/125  "VHAL_LRLDMotorRippleError_flg"
  [VHAL_LRLDMotorRippleError_flg] -> UnitConverter113/1
  zGW_LINDr1/17(VHAL_LRLDValWdwOpened_pct) -> [VHAL_LRLDValWdwOpened_pct]
  UnitConverter114/1 -> bus_creator/126  "VHAL_LRLDValWdwOpened_pct"
  [VHAL_LRLDValWdwOpened_pct] -> UnitConverter114/1
  zGW_LINDr1/18(VHAL_LRRDMotorRelayError_flg) -> [VHAL_LRRDMotorRelayError_flg]
  UnitConverter115/1 -> bus_creator/127  "VHAL_LRRDMotorRelayError_flg"
  [VHAL_LRRDMotorRelayError_flg] -> UnitConverter115/1
  zGW_LINDr1/19(VHAL_LRRDMotorRippleError_flg) -> [VHAL_LRRDMotorRippleError_flg]
  UnitConverter116/1 -> bus_creator/128  "VHAL_LRRDMotorRippleError_flg"
  [VHAL_LRRDMotorRippleError_flg] -> UnitConverter116/1
  zGW_LINDr1/20(VHAL_LRRDValWdwOpened_pct) -> [VHAL_LRRDValWdwOpened_pct]
  UnitConverter117/1 -> bus_creator/129  "VHAL_LRRDValWdwOpened_pct"
  [VHAL_LRRDValWdwOpened_pct] -> UnitConverter117/1
  zGW_LINDr1/21(VHAL_RAPWL01LINResponseError_flg) -> [VHAL_RAPWL01LINResponseError_flg]
  UnitConverter118/1 -> bus_creator/130  "VHAL_RAPWL01LINResponseError_flg"
  [VHAL_RAPWL01LINResponseError_flg] -> UnitConverter118/1
  zGW_LINDr1/22(VHAL_RLSLampSta_flg) -> [VHAL_RLSLampSta_flg]
  UnitConverter119/1 -> bus_creator/131  "VHAL_RLSLampSta_flg"
  [VHAL_RLSLampSta_flg] -> UnitConverter119/1
  zGW_LINDr1/23(VHAL_RLSRainSnrWiperCmd_enum) -> [VHAL_RLSRainSnrWiperCmd_enum]
  UnitConverter120/1 -> bus_creator/132  "VHAL_RLSRainSnrWiperCmd_enum"
  [VHAL_RLSRainSnrWiperCmd_enum] -> UnitConverter120/1
  zGW_LINDr1/24(VHAL_SWCACCSta_flg) -> [VHAL_SWCACCSta_flg]
  UnitConverter121/1 -> bus_creator/133  "VHAL_SWCACCSta_flg"
  [VHAL_SWCACCSta_flg] -> UnitConverter121/1
  zGW_LINDr1/25(VHAL_SWCCANCELSta_flg) -> [VHAL_SWCCANCELSta_flg]
  UnitConverter122/1 -> bus_creator/134  "VHAL_SWCCANCELSta_flg"
  [VHAL_SWCCANCELSta_flg] -> UnitConverter122/1
  zGW_LINDr1/26(VHAL_SWCDistanceSta_flg) -> [VHAL_SWCDistanceSta_flg]
  UnitConverter123/1 -> bus_creator/135  "VHAL_SWCDistanceSta_flg"
  [VHAL_SWCDistanceSta_flg] -> UnitConverter123/1
  zGW_LINDr1/27(VHAL_SWCDownSta_flg) -> [VHAL_SWCDownSta_flg]
  UnitConverter124/1 -> bus_creator/136  "VHAL_SWCDownSta_flg"
  [VHAL_SWCDownSta_flg] -> UnitConverter124/1
  zGW_LINDr1/28(VHAL_SWCLKASta_flg) -> [VHAL_SWCLKASta_flg]
  UnitConverter125/1 -> bus_creator/137  "VHAL_SWCLKASta_flg"
  [VHAL_SWCLKASta_flg] -> UnitConverter125/1
  zGW_LINDr1/29(VHAL_SWCLeftSta_flg) -> [VHAL_SWCLeftSta_flg]
  UnitConverter126/1 -> bus_creator/138  "VHAL_SWCLeftSta_flg"
  [VHAL_SWCLeftSta_flg] -> UnitConverter126/1
  zGW_LINDr1/30(VHAL_SWCRegenUp_flg) -> [VHAL_SWCRegenUp_flg]
  UnitConverter127/1 -> bus_creator/139  "VHAL_SWCRegenUp_flg"
  [VHAL_SWCRegenUp_flg] -> UnitConverter127/1
  zGW_LINDr1/31(VHAL_SWCResUpSta_flg) -> [VHAL_SWCResUpSta_flg]
  UnitConverter128/1 -> bus_creator/140  "VHAL_SWCResUpSta_flg"
  [VHAL_SWCResUpSta_flg] -> UnitConverter128/1
  zGW_LINDr1/32(VHAL_SWCRightSta_flg) -> [VHAL_SWCRightSta_flg]
  UnitConverter129/1 -> bus_creator/141  "VHAL_SWCRightSta_flg"
  [VHAL_SWCRightSta_flg] -> UnitConverter129/1
  zGW_LINDr1/33(VHAL_SWCSetdownSta_flg) -> [VHAL_SWCSetdownSta_flg]
  UnitConverter130/1 -> bus_creator/142  "VHAL_SWCSetdownSta_flg"
  [VHAL_SWCSetdownSta_flg] -> UnitConverter130/1
  zGW_LINDr1/34(VHAL_SWCTripSta_flg) -> [VHAL_SWCTripSta_flg]
  UnitConverter131/1 -> bus_creator/143  "VHAL_SWCTripSta_flg"
  [VHAL_SWCTripSta_flg] -> UnitConverter131/1
  zGW_LINDr1/35(VHAL_SWCUndefinedSta_flg) -> [VHAL_SWCUndefinedSta_flg]
  UnitConverter132/1 -> bus_creator/144  "VHAL_SWCUndefinedSta_flg"
  [VHAL_SWCUndefinedSta_flg] -> UnitConverter132/1
  zGW_LINDr1/36(VHAL_SWCUpSta_flg) -> [VHAL_SWCUpSta_flg]
  UnitConverter133/1 -> bus_creator/145  "VHAL_SWCUpSta_flg"
  [VHAL_SWCUpSta_flg] -> UnitConverter133/1
  zGW_LINDr1/37(VHAL_SWCVRSta_flg) -> [VHAL_SWCVRSta_flg]
  UnitConverter134/1 -> bus_creator/146  "VHAL_SWCVRSta_flg"
  [VHAL_SWCVRSta_flg] -> UnitConverter134/1
  zGW_LINDr1/38(VHAL_SWCmodeSta_flg) -> [VHAL_SWCmodeSta_flg]
  UnitConverter135/1 -> bus_creator/147  "VHAL_SWCmodeSta_flg"
  [VHAL_SWCmodeSta_flg] -> UnitConverter135/1

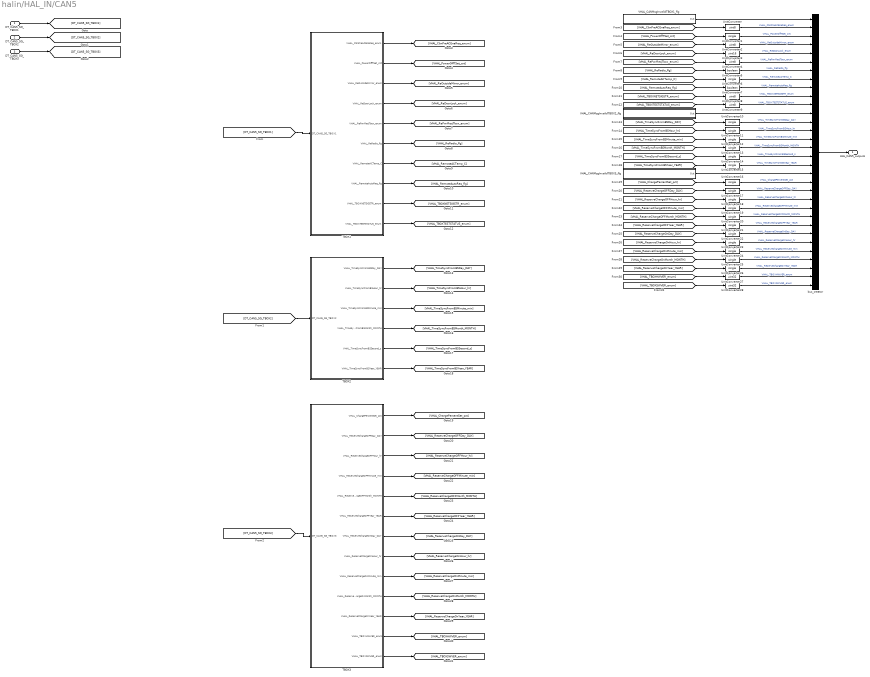
== system halin/HAL_IN/CAN5 ==
  DT_CAN5_SG_TBOX1 : Inport
  DT_CAN5_SG_TBOX2 : Inport  Port=2
  DT_CAN5_SG_TBOX3 : Inport  Port=3
  TBOX1 : Subsystem
  TBOX2 : Subsystem
  TBOX3 : Subsystem
  UnitConverter{,2,4,8..9} (5 alike) : DataTypeConversion  OutDataTypeStr=uint8
  UnitConverter{1,6,10..26} (19 alike) : DataTypeConversion  OutDataTypeStr=single
  UnitConverter27 : DataTypeConversion  OutDataTypeStr=uint32
  UnitConverter28 : DataTypeConversion  OutDataTypeStr=uint32
  UnitConverter3 : DataTypeConversion  OutDataTypeStr=uint16
  UnitConverter5 : DataTypeConversion  OutDataTypeStr=boolean
  UnitConverter7 : DataTypeConversion  OutDataTypeStr=boolean
  VHAL_CANMsgInvalidTBOX1_flg : Subsystem  AncestorBlock=FVT_lib/hal/MsgTimeoutJudge_CAN_AUTOSAR
      mask help: MeasumentTrigerEvent
      mask Display: fprintf('MsgTimeoutJudge_CAN\nAUTOSAR');
  VHAL_CANMsgInvalidTBOX2_flg : Subsystem  AncestorBlock=FVT_lib/hal/MsgTimeoutJudge_CAN_AUTOSAR
      mask help: MeasumentTrigerEvent
      mask Display: fprintf('MsgTimeoutJudge_CAN\nAUTOSAR');
  VHAL_CANMsgInvalidTBOX3_flg : Subsystem  AncestorBlock=FVT_lib/hal/MsgTimeoutJudge_CAN_AUTOSAR
      mask help: MeasumentTrigerEvent
      mask Display: fprintf('MsgTimeoutJudge_CAN\nAUTOSAR');
  bus_creator : BusCreator  Inputs=32
  HAL_CAN5_outputs : Outport
  wires:
  DT_CAN5_SG_TBOX1/1 -> [DT_CAN5_SG_TBOX1]
  DT_CAN5_SG_TBOX2/1 -> [DT_CAN5_SG_TBOX2]
  DT_CAN5_SG_TBOX3/1 -> [DT_CAN5_SG_TBOX3]
  [DT_CAN5_SG_TBOX1] -> TBOX1/1(DT_CAN5_SG_TBOX1)
  [DT_CAN5_SG_TBOX2] -> TBOX2/1(DT_CAN5_SG_TBOX2)
  [DT_CAN5_SG_TBOX3] -> TBOX3/1(DT_CAN5_SG_TBOX3)
  bus_creator/1 -> HAL_CAN5_outputs/1
  VHAL_CANMsgInvalidTBOX1_flg/1(Out) -> bus_creator/1
  TBOX1/1(VHAL_CbnPreACEnaReq_enum) -> [VHAL_CbnPreACEnaReq_enum]
  UnitConverter/1 -> bus_creator/2  "VHAL_CbnPreACEnaReq_enum"
  [VHAL_CbnPreACEnaReq_enum] -> UnitConverter/1
  TBOX1/2(VHAL_PowerOffTSet_cnt) -> [VHAL_PowerOffTSet_cnt]
  UnitConverter1/1 -> bus_creator/3  "VHAL_PowerOffTSet_cnt"
  [VHAL_PowerOffTSet_cnt] -> UnitConverter1/1
  TBOX1/3(VHAL_ReOutsideMirror_enum) -> [VHAL_ReOutsideMirror_enum]
  UnitConverter2/1 -> bus_creator/4  "VHAL_ReOutsideMirror_enum"
  [VHAL_ReOutsideMirror_enum] -> UnitConverter2/1
  TBOX1/4(VHAL_ReDoorLock_enum) -> [VHAL_ReDoorLock_enum]
  UnitConverter3/1 -> bus_creator/5  "VHAL_ReDoorLock_enum"
  [VHAL_ReDoorLock_enum] -> UnitConverter3/1
  TBOX1/5(VHAL_RePwrReqTbox_enum) -> [VHAL_RePwrReqTbox_enum]
  UnitConverter4/1 -> bus_creator/6  "VHAL_RePwrReqTbox_enum"
  [VHAL_RePwrReqTbox_enum] -> UnitConverter4/1
  TBOX1/6(VHAL_ReRadio_flg) -> [VHAL_ReRadio_flg]
  UnitConverter5/1 -> bus_creator/7  "VHAL_ReRadio_flg"
  [VHAL_ReRadio_flg] -> UnitConverter5/1
  TBOX1/7(VHAL_RemoteACTemp_C) -> [VHAL_RemoteACTemp_C]
  UnitConverter6/1 -> bus_creator/8  "VHAL_RemoteACTemp_C"
  [VHAL_RemoteACTemp_C] -> UnitConverter6/1
  TBOX1/8(VHAL_RemoteAutoReq_flg) -> [VHAL_RemoteAutoReq_flg]
  UnitConverter7/1 -> bus_creator/9  "VHAL_RemoteAutoReq_flg"
  [VHAL_RemoteAutoReq_flg] -> UnitConverter7/1
  TBOX1/9(VHAL_TBOXNETSIGSTR_enum) -> [VHAL_TBOXNETSIGSTR_enum]
  UnitConverter8/1 -> bus_creator/10  "VHAL_TBOXNETSIGSTR_enum"
  [VHAL_TBOXNETSIGSTR_enum] -> UnitConverter8/1
  TBOX1/10(VHAL_TBOXTESTSTATUS_enum) -> [VHAL_TBOXTESTSTATUS_enum]
  UnitConverter9/1 -> bus_creator/11  "VHAL_TBOXTESTSTATUS_enum"
  [VHAL_TBOXTESTSTATUS_enum] -> UnitConverter9/1
  VHAL_CANMsgInvalidTBOX2_flg/1(Out) -> bus_creator/12
  TBOX2/1(VHAL_TimeSyncFromBSDay_DAY) -> [VHAL_TimeSyncFromBSDay_DAY]
  UnitConverter10/1 -> bus_creator/13  "VHAL_TimeSyncFromBSDay_DAY"
  [VHAL_TimeSyncFromBSDay_DAY] -> UnitConverter10/1
  TBOX2/2(VHAL_TimeSyncFromBSHour_hr) -> [VHAL_TimeSyncFromBSHour_hr]
  UnitConverter11/1 -> bus_creator/14  "VHAL_TimeSyncFromBSHour_hr"
  [VHAL_TimeSyncFromBSHour_hr] -> UnitConverter11/1
  TBOX2/3(VHAL_TimeSyncFromBSMinute_min) -> [VHAL_TimeSyncFromBSMinute_min]
  UnitConverter12/1 -> bus_creator/15  "VHAL_TimeSyncFromBSMinute_min"
  [VHAL_TimeSyncFromBSMinute_min] -> UnitConverter12/1
  TBOX2/4(VHAL_TimeSyncFromBSMonth_MONTH) -> [VHAL_TimeSyncFromBSMonth_MONTH]
  UnitConverter13/1 -> bus_creator/16  "VHAL_TimeSyncFromBSMonth_MONTH"
  [VHAL_TimeSyncFromBSMonth_MONTH] -> UnitConverter13/1
  TBOX2/5(VHAL_TimeSyncFromBSSecond_s) -> [VHAL_TimeSyncFromBSSecond_s]
  UnitConverter14/1 -> bus_creator/17  "VHAL_TimeSyncFromBSSecond_s"
  [VHAL_TimeSyncFromBSSecond_s] -> UnitConverter14/1
  TBOX2/6(VHAL_TimeSyncFromBSYear_YEAR) -> [VHAL_TimeSyncFromBSYear_YEAR]
  UnitConverter15/1 -> bus_creator/18  "VHAL_TimeSyncFromBSYear_YEAR"
  [VHAL_TimeSyncFromBSYear_YEAR] -> UnitConverter15/1
  VHAL_CANMsgInvalidTBOX3_flg/1(Out) -> bus_creator/19
  TBOX3/1(VHAL_ChargePercentSet_pct) -> [VHAL_ChargePercentSet_pct]
  UnitConverter16/1 -> bus_creator/20  "VHAL_ChargePercentSet_pct"
  [VHAL_ChargePercentSet_pct] -> UnitConverter16/1
  TBOX3/2(VHAL_ReserveChargeOFFDay_DAY) -> [VHAL_ReserveChargeOFFDay_DAY]
  UnitConverter17/1 -> bus_creator/21  "VHAL_ReserveChargeOFFDay_DAY"
  [VHAL_ReserveChargeOFFDay_DAY] -> UnitConverter17/1
  TBOX3/3(VHAL_ReserveChargeOFFHour_hr) -> [VHAL_ReserveChargeOFFHour_hr]
  UnitConverter18/1 -> bus_creator/22  "VHAL_ReserveChargeOFFHour_hr"
  [VHAL_ReserveChargeOFFHour_hr] -> UnitConverter18/1
  TBOX3/4(VHAL_ReserveChargeOFFMinute_min) -> [VHAL_ReserveChargeOFFMinute_min]
  UnitConverter19/1 -> bus_creator/23  "VHAL_ReserveChargeOFFMinute_min"
  [VHAL_ReserveChargeOFFMinute_min] -> UnitConverter19/1
  TBOX3/5(VHAL_ReserveChargeOFFMonth_MONTH) -> [VHAL_ReserveChargeOFFMonth_MONTH]
  UnitConverter20/1 -> bus_creator/24  "VHAL_ReserveChargeOFFMonth_MONTH"
  [VHAL_ReserveChargeOFFMonth_MONTH] -> UnitConverter20/1
  TBOX3/6(VHAL_ReserveChargeOFFYear_YEAR) -> [VHAL_ReserveChargeOFFYear_YEAR]
  UnitConverter21/1 -> bus_creator/25  "VHAL_ReserveChargeOFFYear_YEAR"
  [VHAL_ReserveChargeOFFYear_YEAR] -> UnitConverter21/1
  TBOX3/7(VHAL_ReserveChargeOnDay_DAY) -> [VHAL_ReserveChargeOnDay_DAY]
  UnitConverter22/1 -> bus_creator/26  "VHAL_ReserveChargeOnDay_DAY"
  [VHAL_ReserveChargeOnDay_DAY] -> UnitConverter22/1
  TBOX3/8(VHAL_ReserveChargeOnHour_hr) -> [VHAL_ReserveChargeOnHour_hr]
  UnitConverter23/1 -> bus_creator/27  "VHAL_ReserveChargeOnHour_hr"
  [VHAL_ReserveChargeOnHour_hr] -> UnitConverter23/1
  TBOX3/9(VHAL_ReserveChargeOnMinute_min) -> [VHAL_ReserveChargeOnMinute_min]
  UnitConverter24/1 -> bus_creator/28  "VHAL_ReserveChargeOnMinute_min"
  [VHAL_ReserveChargeOnMinute_min] -> UnitConverter24/1
  TBOX3/10(VHAL_ReserveChargeOnMonth_MONTH) -> [VHAL_ReserveChargeOnMonth_MONTH]
  UnitConverter25/1 -> bus_creator/29  "VHAL_ReserveChargeOnMonth_MONTH"
  [VHAL_ReserveChargeOnMonth_MONTH] -> UnitConverter25/1
  TBOX3/11(VHAL_ReserveChargeOnYear_YEAR) -> [VHAL_ReserveChargeOnYear_YEAR]
  UnitConverter26/1 -> bus_creator/30  "VHAL_ReserveChargeOnYear_YEAR"
  [VHAL_ReserveChargeOnYear_YEAR] -> UnitConverter26/1
  TBOX3/12(VHAL_TBOXHWVER_enum) -> [VHAL_TBOXHWVER_enum]
  UnitConverter27/1 -> bus_creator/31  "VHAL_TBOXHWVER_enum"
  [VHAL_TBOXHWVER_enum] -> UnitConverter27/1
  TBOX3/13(VHAL_TBOXSWVER_enum) -> [VHAL_TBOXSWVER_enum]
  UnitConverter28/1 -> bus_creator/32  "VHAL_TBOXSWVER_enum"
  [VHAL_TBOXSWVER_enum] -> UnitConverter28/1

== system halin/HAL_IN/CAN7 ==
  DT_CAN7_SG_Door_Fr1 : Inport
  Door_Fr1 : Subsystem
  UnitConverter : DataTypeConversion  OutDataTypeStr=uint8
  UnitConverter1 : DataTypeConversion  OutDataTypeStr=uint8
  UnitConverter2 : DataTypeConversion  OutDataTypeStr=uint8
  VHAL_CANMsgInvalidDoorFr1_flg : Subsystem  AncestorBlock=FVT_lib/hal/MsgTimeoutJudge_CAN_AUTOSAR
      mask help: MeasumentTrigerEvent
      mask Display: fprintf('MsgTimeoutJudge_CAN\nAUTOSAR');
  bus_creator : BusCreator  Inputs=4
  HAL_CAN7_outputs : Outport
  wires:
  DT_CAN7_SG_Door_Fr1/1 -> [DT_CAN7_SG_Door_Fr1]
  [DT_CAN7_SG_Door_Fr1] -> Door_Fr1/1(DT_CAN7_SG_Door_Fr1)
  bus_creator/1 -> HAL_CAN7_outputs/1
  VHAL_CANMsgInvalidDoorFr1_flg/1(Out) -> bus_creator/1
  Door_Fr1/1(VHAL_DoorFrDoorEmergencysta_enum) -> [VHAL_DoorFrDoorEmergencysta_enum]
  UnitConverter/1 -> bus_creator/2  "VHAL_DoorFrDoorEmergencysta_enum"
  [VHAL_DoorFrDoorEmergencysta_enum] -> UnitConverter/1
  Door_Fr1/2(VHAL_DoorFrDooroperationsta_enum) -> [VHAL_DoorFrDooroperationsta_enum]
  UnitConverter1/1 -> bus_creator/3  "VHAL_DoorFrDooroperationsta_enum"
  [VHAL_DoorFrDooroperationsta_enum] -> UnitConverter1/1
  Door_Fr1/3(VHAL_DoorFrDoorpositionsta_enum) -> [VHAL_DoorFrDoorpositionsta_enum]
  UnitConverter2/1 -> bus_creator/4  "VHAL_DoorFrDoorpositionsta_enum"
  [VHAL_DoorFrDoorpositionsta_enum] -> UnitConverter2/1

== system halin/HAL_IN/CAN1/DCDC_Status_1 ==
  DT_CAN1_SG_DCDC_Status_1 : Inport
  DCDCEnSta : Subsystem
  bus_selector : BusSelector  OutputSignals=CAN1_DCDCEnSta
  VHAL_DCDCEnSta_enum : Outport
  wires:
  DT_CAN1_SG_DCDC_Status_1/1 -> [DT_CAN1_SG_DCDC_Status_1]
  [DT_CAN1_SG_DCDC_Status_1] -> bus_selector/1
  bus_selector/1 -> DCDCEnSta/1(DCDCEnSta)  "<CAN1_DCDCEnSta>"
  DCDCEnSta/1(VHAL_DCDCEnSta_enum) -> VHAL_DCDCEnSta_enum/1

== system halin/HAL_IN/CAN1/DCDC_Status_2 ==
  DT_CAN1_SG_DCDC_Status_2 : Inport
  DCDCOutVol : Subsystem
  bus_selector : BusSelector  OutputSignals=CAN1_DCDCOutVol
  VHAL_DCDCOutVol_V : Outport
  wires:
  DT_CAN1_SG_DCDC_Status_2/1 -> [DT_CAN1_SG_DCDC_Status_2]
  [DT_CAN1_SG_DCDC_Status_2] -> bus_selector/1
  bus_selector/1 -> DCDCOutVol/1(DCDCOutVol)  "<CAN1_DCDCOutVol>"
  DCDCOutVol/1(VHAL_DCDCOutVol_V) -> VHAL_DCDCOutVol_V/1

== system halin/HAL_IN/CAN1/EAC_Status_1 ==
  DT_CAN1_SG_EAC_Status_1 : Inport
  EACEnSta : Subsystem
  bus_selector : BusSelector  OutputSignals=CAN1_EACEnSta
  VHAL_EACEnSta_enum : Outport
  wires:
  DT_CAN1_SG_EAC_Status_1/1 -> [DT_CAN1_SG_EAC_Status_1]
  [DT_CAN1_SG_EAC_Status_1] -> bus_selector/1
  bus_selector/1 -> EACEnSta/1(EACEnSta)  "<CAN1_EACEnSta>"
  EACEnSta/1(VHAL_EACEnSta_enum) -> VHAL_EACEnSta_enum/1

== system halin/HAL_IN/CAN1/EBC1 ==
  DT_CAN1_SG_EBC1 : Inport
  ABSFullyOper : Subsystem
  ABSOffroadSw : Subsystem
  ASRBrakeCtrlAtc : Subsystem
  ASREngCtrlAtc : Subsystem
  ASRHillHolderSw : Subsystem
  ASROffroadSw : Subsystem
  ATCASRInfoSig : Subsystem
  AcltrInterlockSw : Subsystem
  AntiLBrakABSAct : Subsystem
  BrakePedalPos : Subsystem
  EBSAmWarnLampSta : Subsystem
  EBSBrakeSw : Subsystem
  EBSRedWarnLampSta : Subsystem
  EngAuxShutdownSw : Subsystem
  EngDerateSw : Subsystem
  EngRetSel : Subsystem
  HaltBrakeSw : Subsystem
  RmAccelEnSw : Subsystem
  SACtrlBrakeCtrl : Subsystem
  TractCtrlOvrSw : Subsystem
  TrailerABSSta : Subsystem
  TrailerABSWarnSig : Subsystem
  bus_selector : BusSelector  OutputSignals=CAN1_ABSFullyOper
  bus_selector1 : BusSelector  OutputSignals=CAN1_ABSOffroadSw
  bus_selector10 : BusSelector  OutputSignals=CAN1_EBSAmWarnLampSta
  bus_selector11 : BusSelector  OutputSignals=CAN1_EBSBrakeSw
  bus_selector12 : BusSelector  OutputSignals=CAN1_EBSRedWarnLampSta
  bus_selector13 : BusSelector  OutputSignals=CAN1_EngAuxShutdownSw
  bus_selector14 : BusSelector  OutputSignals=CAN1_EngDerateSw
  bus_selector15 : BusSelector  OutputSignals=CAN1_EngRetSel
  bus_selector16 : BusSelector  OutputSignals=CAN1_HaltBrakeSw
  bus_selector17 : BusSelector  OutputSignals=CAN1_RmAccelEnSw
  bus_selector18 : BusSelector  OutputSignals=CAN1_SACtrlBrakeCtrl
  bus_selector19 : BusSelector  OutputSignals=CAN1_TractCtrlOvrSw
  bus_selector2 : BusSelector  OutputSignals=CAN1_ASRBrakeCtrlAtc
  bus_selector20 : BusSelector  OutputSignals=CAN1_TrailerABSSta
  bus_selector21 : BusSelector  OutputSignals=CAN1_TrailerABSWarnSig
  bus_selector3 : BusSelector  OutputSignals=CAN1_ASREngCtrlAtc
  bus_selector4 : BusSelector  OutputSignals=CAN1_ASRHillHolderSw
  bus_selector5 : BusSelector  OutputSignals=CAN1_ASROffroadSw
  bus_selector6 : BusSelector  OutputSignals=CAN1_ATCASRInfoSig
  bus_selector7 : BusSelector  OutputSignals=CAN1_AcltrInterlockSw
  bus_selector8 : BusSelector  OutputSignals=CAN1_AntiLBrakABSAct
  bus_selector9 : BusSelector  OutputSignals=CAN1_BrakePedalPos
  VHAL_ABSFullyOper_enum : Outport
  VHAL_ABSOffroadSw_enum : Outport  Port=2
  VHAL_ASRBrakeCtrlAtc_enum : Outport  Port=3
  VHAL_ASREngCtrlAtc_enum : Outport  Port=4
  VHAL_ASRHillHolderSw_enum : Outport  Port=5
  VHAL_ASROffroadSw_enum : Outport  Port=6
  VHAL_ATCASRInfoSig_enum : Outport  Port=7
  VHAL_AcltrInterlockSw_enum : Outport  Port=8
  VHAL_AntiLBrakABSAct_enum : Outport  Port=9
  VHAL_BrakePedalPos_pct : Outport  Port=10
  VHAL_EBSAmWarnLampSta_enum : Outport  Port=11
  VHAL_EBSBrakeSw_enum : Outport  Port=12
  VHAL_EBSRedWarnLampSta_enum : Outport  Port=13
  VHAL_EngAuxShutdownSw_enum : Outport  Port=14
  VHAL_EngDerateSw_enum : Outport  Port=15
  VHAL_EngRetSel_pct : Outport  Port=16
  VHAL_HaltBrakeSw_enum : Outport  Port=17
  VHAL_RmAccelEnSw_enum : Outport  Port=18
  VHAL_SACtrlBrakeCtrl_SA : Outport  Port=19
  VHAL_TractCtrlOvrSw_enum : Outport  Port=20
  VHAL_TrailerABSSta_enum : Outport  Port=21
  VHAL_TrailerABSWarnSig_enum : Outport  Port=22
  wires:
  DT_CAN1_SG_EBC1/1 -> [DT_CAN1_SG_EBC1]
  [DT_CAN1_SG_EBC1] -> bus_selector/1
  bus_selector/1 -> ABSFullyOper/1(ABSFullyOper)  "<CAN1_ABSFullyOper>"
  ABSFullyOper/1(VHAL_ABSFullyOper_enum) -> VHAL_ABSFullyOper_enum/1
  [DT_CAN1_SG_EBC1] -> bus_selector1/1
  bus_selector1/1 -> ABSOffroadSw/1(ABSOffroadSw)  "<CAN1_ABSOffroadSw>"
  ABSOffroadSw/1(VHAL_ABSOffroadSw_enum) -> VHAL_ABSOffroadSw_enum/1
  [DT_CAN1_SG_EBC1] -> bus_selector2/1
  bus_selector2/1 -> ASRBrakeCtrlAtc/1(ASRBrakeCtrlAtc)  "<CAN1_ASRBrakeCtrlAtc>"
  ASRBrakeCtrlAtc/1(VHAL_ASRBrakeCtrlAtc_enum) -> VHAL_ASRBrakeCtrlAtc_enum/1
  [DT_CAN1_SG_EBC1] -> bus_selector3/1
  bus_selector3/1 -> ASREngCtrlAtc/1(ASREngCtrlAtc)  "<CAN1_ASREngCtrlAtc>"
  ASREngCtrlAtc/1(VHAL_ASREngCtrlAtc_enum) -> VHAL_ASREngCtrlAtc_enum/1
  [DT_CAN1_SG_EBC1] -> bus_selector4/1
  bus_selector4/1 -> ASRHillHolderSw/1(ASRHillHolderSw)  "<CAN1_ASRHillHolderSw>"
  ASRHillHolderSw/1(VHAL_ASRHillHolderSw_enum) -> VHAL_ASRHillHolderSw_enum/1
  [DT_CAN1_SG_EBC1] -> bus_selector5/1
  bus_selector5/1 -> ASROffroadSw/1(ASROffroadSw)  "<CAN1_ASROffroadSw>"
  ASROffroadSw/1(VHAL_ASROffroadSw_enum) -> VHAL_ASROffroadSw_enum/1
  [DT_CAN1_SG_EBC1] -> bus_selector6/1
  bus_selector6/1 -> ATCASRInfoSig/1(ATCASRInfoSig)  "<CAN1_ATCASRInfoSig>"
  ATCASRInfoSig/1(VHAL_ATCASRInfoSig_enum) -> VHAL_ATCASRInfoSig_enum/1
  [DT_CAN1_SG_EBC1] -> bus_selector7/1
  bus_selector7/1 -> AcltrInterlockSw/1(AcltrInterlockSw)  "<CAN1_AcltrInterlockSw>"
  AcltrInterlockSw/1(VHAL_AcltrInterlockSw_enum) -> VHAL_AcltrInterlockSw_enum/1
  [DT_CAN1_SG_EBC1] -> bus_selector8/1
  bus_selector8/1 -> AntiLBrakABSAct/1(AntiLBrakABSAct)  "<CAN1_AntiLBrakABSAct>"
  AntiLBrakABSAct/1(VHAL_AntiLBrakABSAct_enum) -> VHAL_AntiLBrakABSAct_enum/1
  [DT_CAN1_SG_EBC1] -> bus_selector9/1
  bus_selector9/1 -> BrakePedalPos/1(BrakePedalPos)  "<CAN1_BrakePedalPos>"
  BrakePedalPos/1(VHAL_BrakePedalPos_pct) -> VHAL_BrakePedalPos_pct/1
  [DT_CAN1_SG_EBC1] -> bus_selector10/1
  bus_selector10/1 -> EBSAmWarnLampSta/1(EBSAmWarnLampSta)  "<CAN1_EBSAmWarnLampSta>"
  EBSAmWarnLampSta/1(VHAL_EBSAmWarnLampSta_enum) -> VHAL_EBSAmWarnLampSta_enum/1
  [DT_CAN1_SG_EBC1] -> bus_selector11/1
  bus_selector11/1 -> EBSBrakeSw/1(EBSBrakeSw)  "<CAN1_EBSBrakeSw>"
  EBSBrakeSw/1(VHAL_EBSBrakeSw_enum) -> VHAL_EBSBrakeSw_enum/1
  [DT_CAN1_SG_EBC1] -> bus_selector12/1
  bus_selector12/1 -> EBSRedWarnLampSta/1(EBSRedWarnLampSta)  "<CAN1_EBSRedWarnLampSta>"
  EBSRedWarnLampSta/1(VHAL_EBSRedWarnLampSta_enum) -> VHAL_EBSRedWarnLampSta_enum/1
  [DT_CAN1_SG_EBC1] -> bus_selector13/1
  bus_selector13/1 -> EngAuxShutdownSw/1(EngAuxShutdownSw)  "<CAN1_EngAuxShutdownSw>"
  EngAuxShutdownSw/1(VHAL_EngAuxShutdownSw_enum) -> VHAL_EngAuxShutdownSw_enum/1
  [DT_CAN1_SG_EBC1] -> bus_selector14/1
  bus_selector14/1 -> EngDerateSw/1(EngDerateSw)  "<CAN1_EngDerateSw>"
  EngDerateSw/1(VHAL_EngDerateSw_enum) -> VHAL_EngDerateSw_enum/1
  [DT_CAN1_SG_EBC1] -> bus_selector15/1
  bus_selector15/1 -> EngRetSel/1(EngRetSel)  "<CAN1_EngRetSel>"
  EngRetSel/1(VHAL_EngRetSel_pct) -> VHAL_EngRetSel_pct/1
  [DT_CAN1_SG_EBC1] -> bus_selector16/1
  bus_selector16/1 -> HaltBrakeSw/1(HaltBrakeSw)  "<CAN1_HaltBrakeSw>"
  HaltBrakeSw/1(VHAL_HaltBrakeSw_enum) -> VHAL_HaltBrakeSw_enum/1
  [DT_CAN1_SG_EBC1] -> bus_selector17/1
  bus_selector17/1 -> RmAccelEnSw/1(RmAccelEnSw)  "<CAN1_RmAccelEnSw>"
  RmAccelEnSw/1(VHAL_RmAccelEnSw_enum) -> VHAL_RmAccelEnSw_enum/1
  [DT_CAN1_SG_EBC1] -> bus_selector18/1
  bus_selector18/1 -> SACtrlBrakeCtrl/1(SACtrlBrakeCtrl)  "<CAN1_SACtrlBrakeCtrl>"
  SACtrlBrakeCtrl/1(VHAL_SACtrlBrakeCtrl_SA) -> VHAL_SACtrlBrakeCtrl_SA/1
  [DT_CAN1_SG_EBC1] -> bus_selector19/1
  bus_selector19/1 -> TractCtrlOvrSw/1(TractCtrlOvrSw)  "<CAN1_TractCtrlOvrSw>"
  TractCtrlOvrSw/1(VHAL_TractCtrlOvrSw_enum) -> VHAL_TractCtrlOvrSw_enum/1
  [DT_CAN1_SG_EBC1] -> bus_selector20/1
  bus_selector20/1 -> TrailerABSSta/1(TrailerABSSta)  "<CAN1_TrailerABSSta>"
  TrailerABSSta/1(VHAL_TrailerABSSta_enum) -> VHAL_TrailerABSSta_enum/1
  [DT_CAN1_SG_EBC1] -> bus_selector21/1
  bus_selector21/1 -> TrailerABSWarnSig/1(TrailerABSWarnSig)  "<CAN1_TrailerABSWarnSig>"
  TrailerABSWarnSig/1(VHAL_TrailerABSWarnSig_enum) -> VHAL_TrailerABSWarnSig_enum/1

== system halin/HAL_IN/CAN1/EBC2 ==
  DT_CAN1_SG_EBC2 : Inport
  FASpeed : Subsystem
  RelaSpdFALWheel : Subsystem
  RelaSpdFARWheel : Subsystem
  bus_selector : BusSelector  OutputSignals=CAN1_FASpeed
  bus_selector1 : BusSelector  OutputSignals=CAN1_RelaSpdFALWheel
  bus_selector2 : BusSelector  OutputSignals=CAN1_RelaSpdFARWheel
  VHAL_FASpeed_kph : Outport
  VHAL_RelaSpdFALWheel_kph : Outport  Port=2
  VHAL_RelaSpdFARWheel_kph : Outport  Port=3
  wires:
  DT_CAN1_SG_EBC2/1 -> [DT_CAN1_SG_EBC2]
  [DT_CAN1_SG_EBC2] -> bus_selector/1
  bus_selector/1 -> FASpeed/1(FASpeed)  "<CAN1_FASpeed>"
  FASpeed/1(VHAL_FASpeed_kph) -> VHAL_FASpeed_kph/1
  [DT_CAN1_SG_EBC2] -> bus_selector1/1
  bus_selector1/1 -> RelaSpdFALWheel/1(RelaSpdFALWheel)  "<CAN1_RelaSpdFALWheel>"
  RelaSpdFALWheel/1(VHAL_RelaSpdFALWheel_kph) -> VHAL_RelaSpdFALWheel_kph/1
  [DT_CAN1_SG_EBC2] -> bus_selector2/1
  bus_selector2/1 -> RelaSpdFARWheel/1(RelaSpdFARWheel)  "<CAN1_RelaSpdFARWheel>"
  RelaSpdFARWheel/1(VHAL_RelaSpdFARWheel_kph) -> VHAL_RelaSpdFARWheel_kph/1
